simulink model "meas_TF_tcoil"  (R2023b)
settings: Solver=ode15s  StartTime=0.0  StopTime=1e-3  RelTol=1e-3
libraries: fl_lib x6, ee_lib x4, nesl_utility x3, dspfdesign x3, simulink_extras x2, dspsrcs4 x1, dspspect3 x1, dspmathops x1
settings Model: Creator=kschutz  LastModifiedBy=kschutz

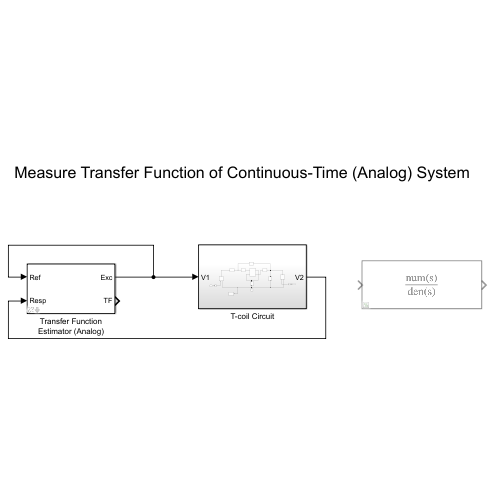
[thumbnail: Simulink's stored preview of the top-level diagram]
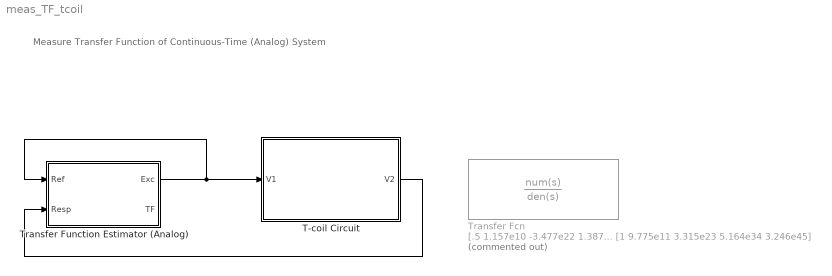
== system meas_TF_tcoil ==
  note: Measure Transfer Function of Continuous-Time (Analog) System
  T-coil Circuit : Subsystem
  Transfer Fcn : TransferFcn  Commented=on  Numerator=[.5 1.157e10 -3.477e22 1.387e32 1.531e45]  Denominator=[1 9.775e11 3.315e23 5.164e34 3.246e45]
  Transfer Function Estimator (Analog) : Subsystem  mask(Baseband Analog Transfer Function Estimator){BW=200e9, Nfft=1000, Navg=100, HoldOff=.1e-9}
      mask prompts: BW "Bandwidth"; Nfft "FFT size"; Navg "Number of Averages"; HoldOff "Hold Off (seconds)"
      mask init:
      | % Select subset of FFT bins that are not aliased
      | % for output and display purposes.
      | % Said subset is based on the oversampling factor.
      | % Here we use a 2.56x oversampling factor.
      | % For example, for a 1024 point FFT size, the relatively
      | % alias free FFT bins would be bins 1 to 401.
      | % floor(1024/2.56) + 1 = 401.
      | OSR = 2.56;
      | AliasFree = floor(Nfft/OSR) + 1;
  wires:
  Transfer Function Estimator (Analog)/1(Exc) -> T-coil Circuit/1(V1), Transfer Function Estimator (Analog)/1(Ref)
  T-coil Circuit/1(V2) -> Transfer Function Estimator (Analog)/2(Resp)

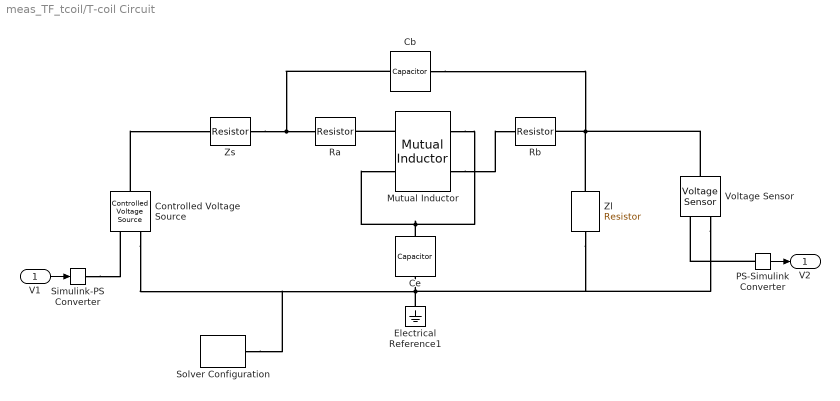
== system meas_TF_tcoil/T-coil Circuit ==
  V1 : Inport
  Cb : ee_lib/Passive/Capacitor  cap_option=ee.enum.passive.capacitor.capOption.const  c=15e-15 F  Cvec=[1e-05, 1e-06] F  Vvec=[0, 10] V  CV_table_symmetry=1  f_vec=[1, 10] kHz  DFext_vec=[.8, 1.2]  enable_C_tol=0  averaging_period=0 s  C_tol=5  tol_distribution=1  nSigma=4  r=1e-6 Ohm  g=0 1/Ohm  enable_operating_limits=0  operating_limit_action=2  max_working_voltage_range=[-25, 25] V  power_rating=1 W  enable_faults=ee.enum.enable.no  fault_action=simscape.enum.assert.action.none  Cscale_faulted=100  R_faulted=1e-3 Ohm  G_faulted=0 1/Ohm  tau_fault=1e-3 s  fault_trigger=ee.enum.faults.faultTrigger.temporal  t_fault=1 s  max_permissible_voltage_range=[-100, 100] V  t_fail_on_voltage=1 s  i_specify=off  i_priority=None  i=0 A  i_nominal_specify=off  i_nominal_unit=A  i_nominal_value=1  v_specify=off  v_priority=None  v=0 V  v_nominal_specify=off  v_nominal_unit=V  v_nominal_value=1  vc_specify=off  vc_priority=High  vc=0 V  vc_nominal_specify=off  vc_nominal_unit=V  vc_nominal_value=1
      settings: AttributesFormatString=%<c> %<c_unit>
  Ce : ee_lib/Passive/Capacitor  cap_option=ee.enum.passive.capacitor.capOption.const  c=300e-15 F  Cvec=[1e-05, 1e-06] F  Vvec=[0, 10] V  CV_table_symmetry=1  f_vec=[1, 10] kHz  DFext_vec=[.8, 1.2]  enable_C_tol=0  averaging_period=0 s  C_tol=5  tol_distribution=1  nSigma=4  r=1e-6 Ohm  g=0 1/Ohm  enable_operating_limits=0  operating_limit_action=2  max_working_voltage_range=[-25, 25] V  power_rating=1 W  enable_faults=ee.enum.enable.no  fault_action=simscape.enum.assert.action.none  Cscale_faulted=100  R_faulted=1e-3 Ohm  G_faulted=0 1/Ohm  tau_fault=1e-3 s  fault_trigger=ee.enum.faults.faultTrigger.temporal  t_fault=1 s  max_permissible_voltage_range=[-100, 100] V  t_fail_on_voltage=1 s  i_specify=off  i_priority=None  i=0 A  i_nominal_specify=off  i_nominal_unit=A  i_nominal_value=1  v_specify=off  v_priority=None  v=0 V  v_nominal_specify=off  v_nominal_unit=V  v_nominal_value=1  vc_specify=off  vc_priority=High  vc=0 V  vc_nominal_specify=off  vc_nominal_unit=V  vc_nominal_value=1
      settings: AttributesFormatString=%<c> %<c_unit>
  Controlled Voltage Source : fl_lib/Electrical/Electrical Sources/Controlled Voltage Source
  Electrical Reference1 : fl_lib/Electrical/Electrical Elements/Electrical Reference
  Mutual Inductor : fl_lib/Electrical/Electrical Elements/Mutual Inductor  L1=360e-12 H  L2=240e-12 H  k=.4  i1_specify=off  i1_priority=High  i1=0 A  i1_nominal_specify=off  i1_nominal_unit=A  i1_nominal_value=1  i2_specify=off  i2_priority=High  i2=0 A  i2_nominal_specify=off  i2_nominal_unit=A  i2_nominal_value=1  v1_specify=off  v1_priority=None  v1=0 V  v1_nominal_specify=off  v1_nominal_unit=V  v1_nominal_value=1  v2_specify=off  v2_priority=None  v2=0 V  v2_nominal_specify=off  v2_nominal_unit=V  v2_nominal_value=1
      settings: InternalSimscapePortConfiguration="{\"Bottom\":[],\"Left\":[{\"id\":\"p1\",\"label\":\"1+\",\"type\":\"foundation.electrical.electrical\"},{\"id\":\"n1\",\"label\":\"1-\",\"type\":\"foundation.electrical.electrical\"}],\"Right\":[{\"id\":\"p2\",\"label\":\"2+\",\"type\":\"foundation.electrical.electrical\"},{\"id\":\"n2\",\"label\":\"2-\",\"type\":\"foundation.electrical.electrical\"}],\"Top\":[]}"
      settings: AttributesFormatString=|
      | %<L1> %<L1_unit>
      | %<L2> %<L2_unit>
  PS-Simulink Converter : nesl_utility/PS-Simulink Converter  PhysicalDomain=network_engine_domain  SubClassName=ps_output  LeftPortType=input  RightPortType=output  PseudoPeriodic=off  Frequencies=[]  VectorFormat=inherit  Unit=inherit  AffineConversion=off
  Ra : ee_lib/Passive/Resistor  R=4 Ohm  enable_R_tol=0  R_tol=5  tol_distribution=1  nSigma=4  enable_operating_limits=0  operating_limit_action=2  power_rating=1 W  max_working_voltage=100 V  enable_faults=ee.enum.enable.no  fault_action=simscape.enum.assert.action.none  R_faulted=inf Ohm  fault_trigger=ee.enum.faults.faultTrigger.temporal  t_fault=1 s  max_permissible_current=1 A  t_fail_on_current=1 s  noise_mode=0  Tdevice=25 degC  sample_time=1e-3 s  repeatability=1  user_seed=0  auto_seed=1196140742  faulted_specify=off  faulted_priority=None  faulted=0  power_derating_T1=70 degC  power_derating_T2=155 degC  operating_temperature_range_vec=[-50, 150] degC  alpha=3.93e-3 1/K  Tmeas=25 degC  thermal_mass=100 J/K  temperature_specify=off  temperature_priority=High  temperature=298.15 K  temperature_nominal_specify=off  temperature_nominal_unit=K  temperature_nominal_value=1
      settings: AttributesFormatString=%<R> %<R_unit>
  Rb : ee_lib/Passive/Resistor  R=2 Ohm  enable_R_tol=0  R_tol=5  tol_distribution=1  nSigma=4  enable_operating_limits=0  operating_limit_action=2  power_rating=1 W  max_working_voltage=100 V  enable_faults=ee.enum.enable.no  fault_action=simscape.enum.assert.action.none  R_faulted=inf Ohm  fault_trigger=ee.enum.faults.faultTrigger.temporal  t_fault=1 s  max_permissible_current=1 A  t_fail_on_current=1 s  noise_mode=0  Tdevice=25 degC  sample_time=1e-3 s  repeatability=1  user_seed=0  auto_seed=2348838240  faulted_specify=off  faulted_priority=None  faulted=0  power_derating_T1=70 degC  power_derating_T2=155 degC  operating_temperature_range_vec=[-50, 150] degC  alpha=3.93e-3 1/K  Tmeas=25 degC  thermal_mass=100 J/K  temperature_specify=off  temperature_priority=High  temperature=298.15 K  temperature_nominal_specify=off  temperature_nominal_unit=K  temperature_nominal_value=1
      settings: AttributesFormatString=%<R> %<R_unit>
  Simulink-PS Converter : nesl_utility/Simulink-PS Converter  PhysicalDomain=network_engine_domain  SubClassName=ps_input  LeftPortType=input  RightPortType=output  PseudoPeriodic=off  Frequencies=[]  NoiseDistribution=none  NoiseParameters=[]  Unit=1  AffineConversion=off  FilteringAndDerivatives=provide  SimscapeFilterOrder=1  InputFilterTimeConstant=0.001  UdotUserProvided=0
  Solver Configuration : nesl_utility/Solver Configuration  PhysicalDomain=network_engine_domain  SubClassName=solver  LeftPortType=input  RightPortType=generic  Tones=[]  Harmonics=[]  SimulateNoise=off  Profile=off  UseLocalSampling=off  EnableSwitchedLinearOptims=on  FrequencyDomain=off  UseCCode=off  RelTol=0.001  AbsTol=0.001  MinStep=1e-09  ToWorkspace=off  RevertToSquareIcSolve=off  NumHomotopyIterations=100  PhasorMode=off  PhasorModeNumHarmonics=1  ConsistencySolver=NEWTON_XTOL_AFTER_FTOL  IndexReductionMethod=DerivativeReplacement  DoDC=off  ResidualTolerance=1e-09  ConsistencyTolSource=GLOBAL  ConsistencyAbsTol=0.001  ConsistencyRelTol=0.001  ConsistencyTolFactor=0.001  UseLocalSolver=off  LocalSolverChoice=NE_BACKWARD_EULER_ADVANCER  ResolveIndetEquations=on  FunctionEvalNumThread=1  LocalSolverSampleTime=0.001  DoFixedCost=off  MaxNonlinIter=3  MaxModeIter=2  ComputeImpulses=off  ImpulseIterations=2  LinearAlgebra=auto  LinearAlgebraNumThread=0  EquationFormulation=NE_TIME_EF  DelaysMemoryBudget=1024  AutomaticFiltering=on  FilteringTimeConstant=0.001  PartitionStorageMethod=AS_NEEDED  PartitionMemoryBudget=1024  PartitionMethod=ROBUST  MultibodyUseLocalSolver=off  MultibodyLocalSolverChoice=ODE1  MultibodyLocalSolverSampleTime=0.001
  Voltage Sensor : fl_lib/Electrical/Electrical Sensors/Voltage Sensor
  Zl : fl_lib/Electrical/Electrical Elements/Resistor  R=50 Ohm  i_specify=off  i_priority=None  i=0 A  i_nominal_specify=off  i_nominal_unit=A  i_nominal_value=1  v_specify=off  v_priority=None  v=0 V  v_nominal_specify=off  v_nominal_unit=V  v_nominal_value=1
      settings: AttributesFormatString=%<R> %<R_unit>
  Zs : fl_lib/Electrical/Electrical Elements/Resistor  R=50 Ohm  i_specify=off  i_priority=None  i=0 A  i_nominal_specify=off  i_nominal_unit=A  i_nominal_value=1  v_specify=off  v_priority=None  v=0 V  v_nominal_specify=off  v_nominal_unit=V  v_nominal_value=1
      settings: AttributesFormatString=%<R> %<R_unit>
  V2 : Outport
  wires:
  PS-Simulink Converter/1 -> V2/1
  V1/1 -> Simulink-PS Converter/1
  connections:
  Simulink-PS Converter/RConn1 -- Controlled Voltage Source/RConn1
  Zs/RConn1 -- Cb/RConn1 -- Ra/LConn1
  Ce/RConn1 -- Solver Configuration/RConn1 -- Controlled Voltage Source/RConn2 -- Voltage Sensor/RConn2 -- Zl/RConn1 -- Electrical Reference1/LConn1
  PS-Simulink Converter/LConn1 -- Voltage Sensor/RConn1
  Ce/LConn1 -- Mutual Inductor/RConn1 -- Mutual Inductor/LConn2
  Controlled Voltage Source/LConn1 -- Zs/LConn1
  Zl/LConn1 -- Voltage Sensor/LConn1 -- Cb/LConn1 -- Rb/RConn1
  Mutual Inductor/RConn2 -- Rb/LConn1
  Mutual Inductor/LConn1 -- Ra/RConn1

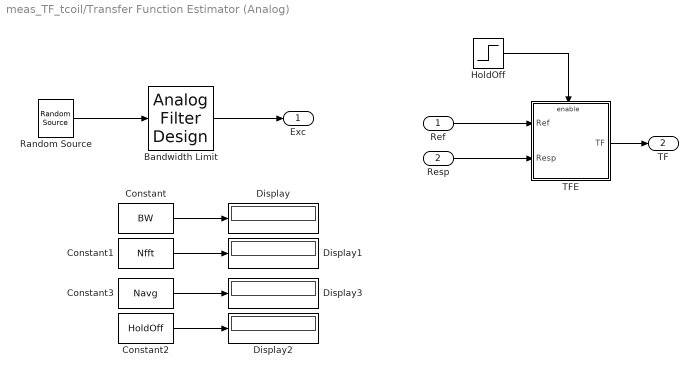
== system meas_TF_tcoil/Transfer Function Estimator (Analog) ==
  Ref : Inport
  Resp : Inport  Port=2
  Bandwidth Limit : dspfdesign/Analog Filter Design  method=Elliptic  filttype=Lowpass  N=8  Wlo=2*pi*BW  Whi=80  Rp=2  Rs=120
  Constant : Constant  Value=BW
  Constant1 : Constant  Value=Nfft
  Constant2 : Constant  Value=HoldOff
  Constant3 : Constant  Value=Navg
  Display{,1..3} (4 alike) : Display
  HoldOff : Step  Time=HoldOff  SampleTime=0
  Random Source : dspsrcs4/Random Source  SrcType=Uniform  NormMethod=Ziggurat  CltLength=12  MinVal=0  MaxVal=1  MeanVal=0  VarVal=1  RepMode=Specify seed  rawSeed=1  IsInherit=off  SampMode=Discrete  SampTime=1/(2.56*BW)  SampFrame=1  DataType=Double  OutComplex=Real  OutputFrames=off
  TFE : Subsystem
  Exc : Outport
  TF : Outport  Port=2
  wires:
  TFE/1(TF) -> TF/1
  Bandwidth Limit/1 -> Exc/1
  Random Source/1 -> Bandwidth Limit/1
  Constant1/1 -> Display1/1
  Constant2/1 -> Display2/1
  Constant/1 -> Display/1
  Ref/1 -> TFE/1(Ref)
  Resp/1 -> TFE/2(Resp)
  HoldOff/1 -> TFE/Enable
  Constant3/1 -> Display3/1

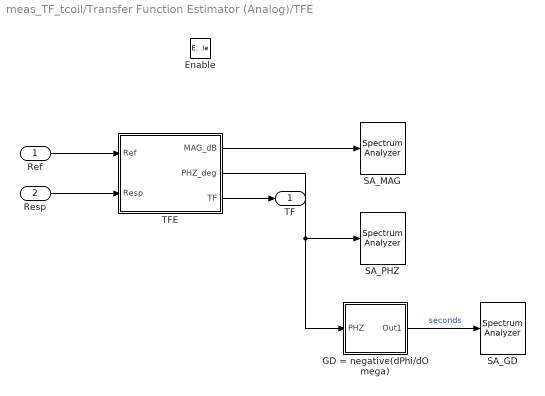
== system meas_TF_tcoil/Transfer Function Estimator (Analog)/TFE ==
  Ref : Inport
  Resp : Inport  Port=2
  Enable : EnablePort
  GD = negative(dPhi/dOmega) : Subsystem
  SA_GD : SpectrumAnalyzer  WindowPosition=[345.000000,56.000000,769.000000,447.000000,]  Visible=on  InputDomain=Frequency  Method=Welch  SampleRateSource=Property  SampleRate=2*BW  PlotAsTwoSidedSpectrum=off  AxesScaling=Manual  InputUnits=dBW  AveragingMethod=Running  SpectrumUnits=dBW  Title=Phase Response  YLabel=Degrees  YLimits=[-1.0584143713275189214,0.1592001832793343008]  IsFrequencyInputMode=1
  SA_MAG : SpectrumAnalyzer  WindowPosition=[1129.000000,656.000000,771.000000,361.000000,]  Visible=on  InputDomain=Frequency  Method=Welch  SampleRateSource=Property  SampleRate=2*BW  PlotAsTwoSidedSpectrum=off  AxesScaling=Manual  InputUnits=dBW  AveragingMethod=Running  SpectrumUnits=dBW  Title=Magnitude Response  YLimits=[-8.12412494,-5.983135]  IsFrequencyInputMode=1
  SA_PHZ : SpectrumAnalyzer  WindowPosition=[1140.000000,132.000000,769.000000,447.000000,]  Visible=on  InputDomain=Frequency  Method=Welch  SampleRateSource=Property  SampleRate=2*BW  PlotAsTwoSidedSpectrum=off  AxesScaling=Manual  InputUnits=dBW  AveragingMethod=Running  SpectrumUnits=dBW  Title=Phase Response  YLabel=Degrees  YLimits=[-224.34422790303892725,224.73028550611314813]  IsFrequencyInputMode=1
  TFE : Subsystem
  TF : Outport
  wires:
  TFE/3(TF) -> TF/1
  Resp/1 -> TFE/2(Resp)
  Ref/1 -> TFE/1(Ref)
  TFE/1(MAG_dB) -> SA_MAG/1
  TFE/2(PHZ_deg) -> GD = negative(dPhi/dOmega)/1(PHZ), SA_PHZ/1
  GD = negative(dPhi/dOmega)/1(Out1) -> SA_GD/1  "seconds"

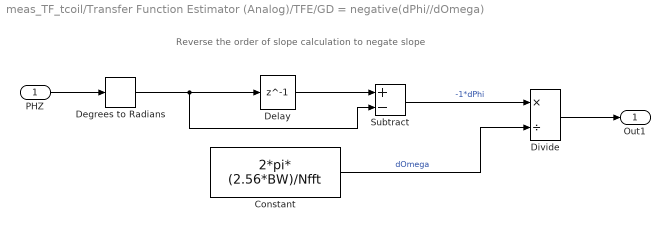
== system meas_TF_tcoil/Transfer Function Estimator (Analog)/TFE/GD = negative(dPhi//dOmega) ==
  note: Reverse the order of slope calculation to negate slope
  PHZ : Inport
  Constant : Constant  Value=2*pi* (2.56*BW)/Nfft
  Degrees to Radians : simulink_extras/Transformations/Degrees to Radians
  Delay : Delay  DelayLength=1  InputProcessing=Columns as channels (frame based)
  Divide : Product  Inputs=*/
  Subtract : Sum  Inputs=+-
  Out1 : Outport  VectorParamsAs1DForOutWhenUnconnected=off
  wires:
  PHZ/1 -> Degrees to Radians/1
  Subtract/1 -> Divide/1  "-1*dPhi"
  Constant/1 -> Divide/2  "dOmega"
  Divide/1 -> Out1/1
  Delay/1 -> Subtract/1
  Degrees to Radians/1 -> Delay/1, Subtract/2

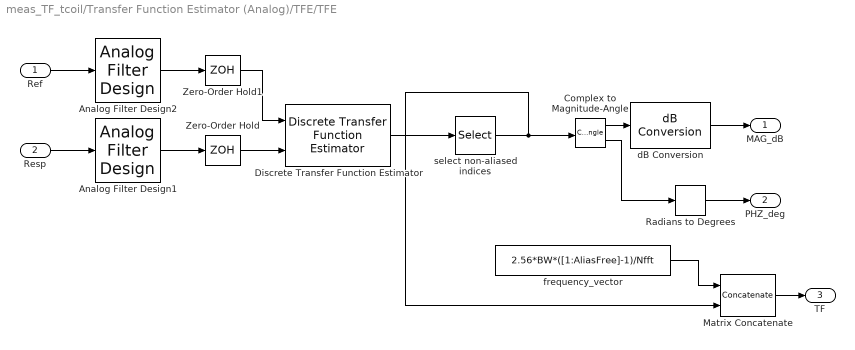
== system meas_TF_tcoil/Transfer Function Estimator (Analog)/TFE/TFE ==
  Ref : Inport
  Resp : Inport  Port=2
  Analog Filter Design1 : dspfdesign/Analog Filter Design  method=Elliptic  filttype=Lowpass  N=8  Wlo=2*pi*BW  Whi=80  Rp=2  Rs=100
  Analog Filter Design2 : dspfdesign/Analog Filter Design  method=Elliptic  filttype=Lowpass  N=8  Wlo=2*pi*BW  Whi=80  Rp=2  Rs=100
  Complex to Magnitude-Angle : ComplexToMagnitudeAngle
  Discrete Transfer Function Estimator : dspspect3/Discrete Transfer Function Estimator  WindowMode=Specify on dialog  WindowLength=Nfft  Overlap=0  AveragingMethod=Running  ForgettingFactorPort=off  ForgettingFactor=0.9  SpectralAverages=Navg  FFTLengthSource=Property  FFTLength=Nfft  Window=Hann  SidelobeAttenuation=60  FrequencyRange=One-sided  OutputCoherence=off  SimulateUsing=Interpreted execution
  Matrix Concatenate : Concatenate  Mode=Multidimensional array  ConcatenateDimension=2
  Radians to Degrees : simulink_extras/Transformations/Radians to Degrees
  Zero-Order Hold : ZeroOrderHold  SampleTime=1/(OSR*BW)
  Zero-Order Hold1 : ZeroOrderHold  SampleTime=1/(OSR*BW)
  dB Conversion : dspmathops/dB Conversion  dBtype=dB  intype=Amplitude  R=1  fuzz=off
  frequency_vector : Constant  Value=2.56*BW*([1:AliasFree]-1)/Nfft
  select non-aliased indices : Selector  NumberOfDimensions=2  InputPortWidth=3  IndexOptions=Index vector (dialog),Select all  Indices=[1:AliasFree ],1  OutputSizes=1,1
  MAG_dB : Outport
  PHZ_deg : Outport  Port=2
  TF : Outport  Port=3
  wires:
  Matrix Concatenate/1 -> TF/1
  select non-aliased indices/1 -> Complex to Magnitude-Angle/1, Matrix Concatenate/2
  frequency_vector/1 -> Matrix Concatenate/1
  Discrete Transfer Function Estimator/1 -> select non-aliased indices/1
  Complex to Magnitude-Angle/2 -> Radians to Degrees/1
  Analog Filter Design1/1 -> Zero-Order Hold/1
  Analog Filter Design2/1 -> Zero-Order Hold1/1
  Radians to Degrees/1 -> PHZ_deg/1
  dB Conversion/1 -> MAG_dB/1
  Resp/1 -> Analog Filter Design1/1
  Zero-Order Hold1/1 -> Discrete Transfer Function Estimator/1
  Ref/1 -> Analog Filter Design2/1
  Complex to Magnitude-Angle/1 -> dB Conversion/1
  Zero-Order Hold/1 -> Discrete Transfer Function Estimator/2
